simulink model "simple_subsystem"  (R2022a)
settings: Solver=VariableStepAuto  StartTime=0.0  StopTime=10.0  RelTol=1e-3
libraries: simulink x1
settings Model: Creator=Home computer  LastModifiedBy=Home computer

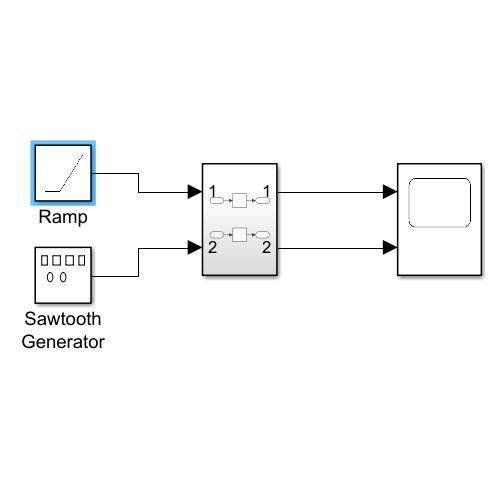
[thumbnail: Simulink's stored preview of the top-level diagram]
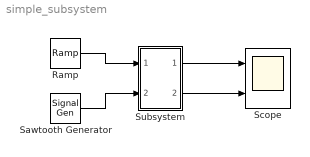
== system simple_subsystem ==
  Ramp : simulink/Sources/Ramp  slope=1  start=0  InitialOutput=0
  Sawtooth Generator : SignalGenerator  WaveForm=sawtooth  Units=rad/sec
  Scope : Scope  NumInputPorts=2
  Subsystem : Subsystem
  wires:
  Ramp/1 -> Subsystem/1(In1)
  Sawtooth Generator/1 -> Subsystem/2(In2)
  Subsystem/1(Out1) -> Scope/1
  Subsystem/2(Out2) -> Scope/2

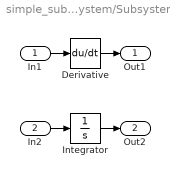
== system simple_subsystem/Subsystem ==
  In1 : Inport
  In2 : Inport  Port=2
  Derivative : Derivative
  Integrator : Integrator
  Out1 : Outport
  Out2 : Outport  Port=2
  wires:
  In1/1 -> Derivative/1
  In2/1 -> Integrator/1
  Integrator/1 -> Out2/1
  Derivative/1 -> Out1/1
